simulink library "UtilLib"  (R2022b)
settings: Solver=VariableStepAuto  StartTime=0.0  StopTime=10.0  RelTol=1e-3
undefined symbols (not defined in the file): ESSettings, simStopTheshold
settings Model: Creator=vd818225  LastModifiedBy=vd818225

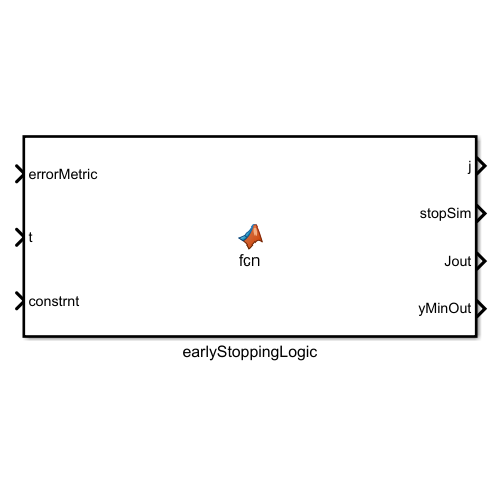
[thumbnail: Simulink's stored preview of the top-level diagram]
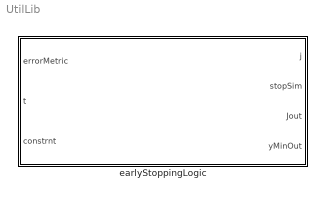
== system UtilLib ==
  earlyStoppingLogic : MATLAB Function  TreatAsAtomicUnit=on

== matlab function UtilLib/earlyStoppingLogic ==
  data: errorMetric input; j output; t input; stopSim output; ESSettings parameter; Jout output; yMinOut output; constrnt input; simStopTheshold parameter
function [j,stopSim,Jout,yMinOut] = fcn(errorMetric,t, ESSettings, constrnt, simStopTheshold)
persistent J
persistent NoOfCalls


tstart = ESSettings.tstart;
tend   = ESSettings.tend;

if isempty(J)
    J = 0;
    NoOfCalls =1;
end
if length(simStopTheshold) == 1
    ymin = simStopTheshold;
else
    ymin = simStopTheshold(NoOfCalls);
end
j = 0;

if tstart <= t && t <= tend
    j = errorMetric;
    NoOfCalls = NoOfCalls +1;
else
    j = 0;
end

J = J + j;

stopSim = false;
if J > ymin
    stopSim = true;
end

Jout = J;
if isinf(ymin)
    ymin = 10^10;
end
yMinOut = ymin;


end
